simulink model "sim_filtros"  (R2021b)
settings: Solver=VariableStepAuto  StartTime=0.0  StopTime=10.0  RelTol=1e-3
settings Model: Creator=osher  LastModifiedBy=osher

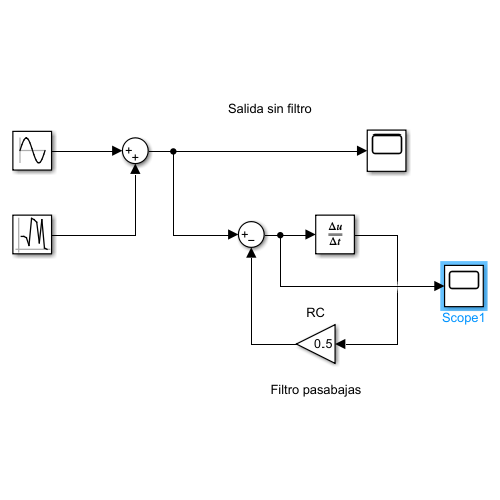
[thumbnail: Simulink's stored preview of the top-level diagram]
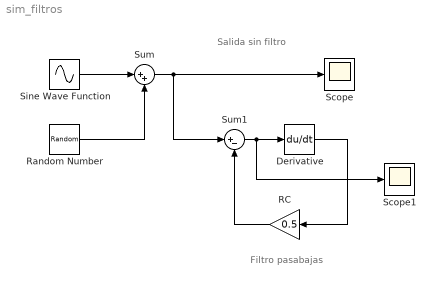
== system sim_filtros ==
  note: Salida sin filtro
  note: Filtro pasabajas
  Derivative : Derivative
  RC : Gain  Gain=0.5
  Random Number : RandomNumber  Variance=3  SampleTime=0.1
  Scope : Scope
  Scope1 : Scope
  Sine Wave Function : Sin  Amplitude=10  Frequency=2  SampleTime=0
  Sum : Sum  Inputs=|++
  Sum1 : Sum  Inputs=|+-
  wires:
  Random Number/1 -> Sum/2
  Sine Wave Function/1 -> Sum/1
  Sum/1 -> Sum1/1, Scope/1
  Sum1/1 -> Scope1/1, Derivative/1
  Derivative/1 -> RC/1
  RC/1 -> Sum1/2
